simulink model "actual_flight"  (R2022a)
settings: Solver=ode4  StartTime=0.0  StopTime=10  FixedStep=0.001  RelTol=1e-3
InitFcn:
  | BeforeSim
undefined symbols (not defined in the file or in its folder): L_ref, S_ref
libraries: simulink_need_slupdate x12
settings Model: Creator=Hans  LastModifiedBy=24659
settings SolverCC: AlgebraicLoopSolver=TrustRegion
settings DataIOCC: ReturnWorkspaceOutputs=off
settings OptimizationCC: LifeSpan=inf
settings DebuggingCC: UnconnectedInputMsg=warning  UnconnectedOutputMsg=warning  UnconnectedLineMsg=warning  SFExecutionAtInitializationDiag=none  SFMachineParentedDataDiag=warning  ArithmeticOperatorsInVariantConditions=warning
settings HardwareCC: ProdBitPerSizeT=32  ProdBitPerPtrDiffT=32  ProdWordSize=32  ProdHWDeviceType=Specified
settings SFSimCC: SimUseLocalCustomCode=off  CustomCodeUndefinedFunction=UseInterfaceOnly
settings RTWCC: RTWUseLocalCustomCode=off
settings CodeAppCC: StateflowObjectComments=on

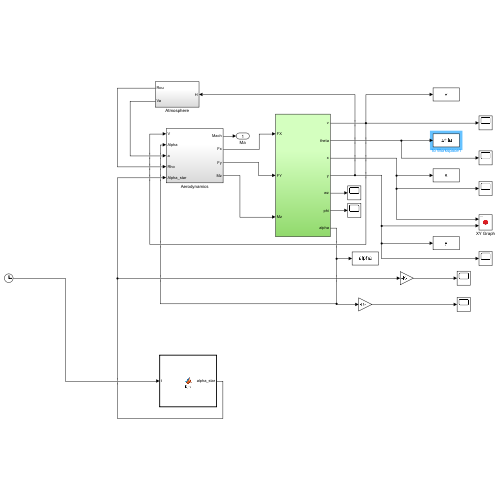
[thumbnail: Simulink's stored preview of the top-level diagram]
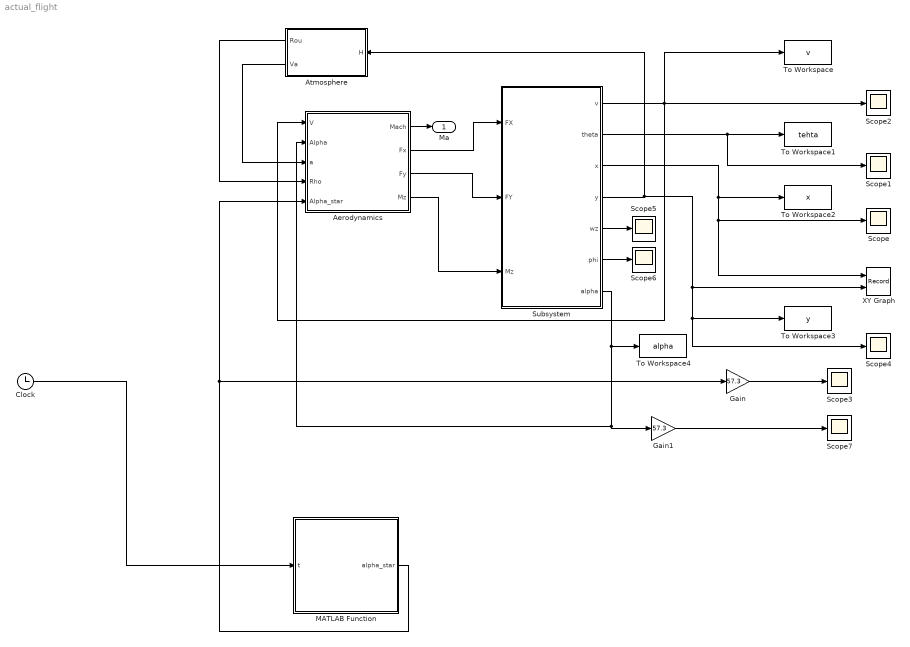
== system actual_flight ==
  Aerodynamics : Subsystem
  Atmosphere : Subsystem
  Clock : Clock
  Gain : Gain  Gain=57.3
  Gain1 : Gain  Gain=57.3
  MATLAB Function : MATLAB Function  TreatAsAtomicUnit=on
  Scope{,1..7} (8 alike) : Scope
  Subsystem : Subsystem
  To Workspace : ToWorkspace  VariableName=v  SaveFormat=Timeseries  SampleTime=-1
  To Workspace1 : ToWorkspace  VariableName=tehta  SaveFormat=Timeseries  SampleTime=-1
  To Workspace2 : ToWorkspace  VariableName=x  SaveFormat=Timeseries  SampleTime=-1
  To Workspace3 : ToWorkspace  VariableName=y  SaveFormat=Timeseries  SampleTime=-1
  To Workspace4 : ToWorkspace  VariableName=alpha  SaveFormat=Timeseries  SampleTime=-1
  XY Graph : Record  FileSettingsInternal="{\"entries\":[{\"content\":{\"excelSettings\":{\"content\":{},\"type\":\"Streamout.ExcelSettings\"}},\"type\":\"Streamout.FileSettingStorage\",\"uuid\":\"ac6b3081-8645-4955-ae6f-fd0c9016351f\"}],\"packageUris\":[\"http://schema.mathworks.com/mf0/streamout_blocks/R2020a\"],\"version\":\"1.0\"}"  Layout=[1 1]  SignalsInternal="{\"entries\":[{\"content\":{\"signals\":[{\"content\":{\"blockPath\":[\"actual_flight/XY Graph\"],\"channel\":[],\"dimensions\":[1],\"domain\":\"actual_flight/XY Graph\",\"lineColor\":\"#a2142f\",\"plots\":[1],\"port\":1,\"sid\":[\"\"],\"signalID\":117,\"signalName\":\"Subsystem:3\"},\"type\":\"RecordBlkView.Signal\",\"uuid\":\"a6b6c65e-2a84-4de5-9352-2b80d4c69f46\"},{\"content\":{\"blockPath\":[\"actual_flight/XY Graph\"],\"channel\":[],\"dimensions\":[1],\"domain\":\"actual_flight/XY Graph\",\"lineColor\":\"#139fff\",\"plots\":[1],\"port\":2,\"sid\":[\"\"],\"signalID\":121,\"signalName\":\"Subsystem:4\"},\"type\":\"RecordBlkView.Signal\",\"uuid\":\"7b7fe503-11ab-499b-9855-293f14eb9002\"}]},\"type\":\"RecordBlkView.InputSignals\",\"uuid\":\"3e16099a-8075-4753-8833-8a8d798b48ad\"}],\"packageUris\":[\"http://schema.mathworks.com/mf0/streamout_blocks/R2020a\"],\"version\":\"1.0\"}"  VisualizationBindings="{\"xyplotplugin\":{\"info\":[{\"series\":[{\"bindingParametersList\":[{\"parameter\":\"X-Axis\",\"signalID\":117,\"signalName\":\"Subsystem:3\"},{\"parameter\":\"Y-Axis\",\"signalID\":121,\"signalName\":\"Subsystem:4\"}],\"seriesID\":55315}],\"subplotID\":1}]}}"  CompatibilityTag=XY  st=-1
  Ma : Outport
  wires:
  Gain/1 -> Scope3/1
  Subsystem/4(y) -> To Workspace3/1, Scope4/1, XY Graph/2, Atmosphere/1(H)
  Subsystem/1(v) -> Aerodynamics/1(V), Scope2/1, To Workspace/1
  Aerodynamics/1(" Mach") -> Ma/1
  Aerodynamics/2(Fx) -> Subsystem/1(FX)
  Atmosphere/1(Rou) -> Aerodynamics/4(Rho)
  Aerodynamics/3(Fy) -> Subsystem/2(FY)
  Atmosphere/2(Va) -> Aerodynamics/3(a)
  Clock/1 -> MATLAB Function/1(t)
  Subsystem/2(theta) -> Scope1/1, To Workspace1/1
  Subsystem/3(x) -> XY Graph/1, Scope/1, To Workspace2/1
  MATLAB Function/1(alpha_star) -> Aerodynamics/5(Alpha_star), Gain/1
  Aerodynamics/4(" Mz") -> Subsystem/3(Mz)
  Subsystem/7(alpha) -> To Workspace4/1, Gain1/1, Aerodynamics/2(Alpha)
  Subsystem/5(wz) -> Scope5/1
  Subsystem/6(phi) -> Scope6/1
  Gain1/1 -> Scope7/1

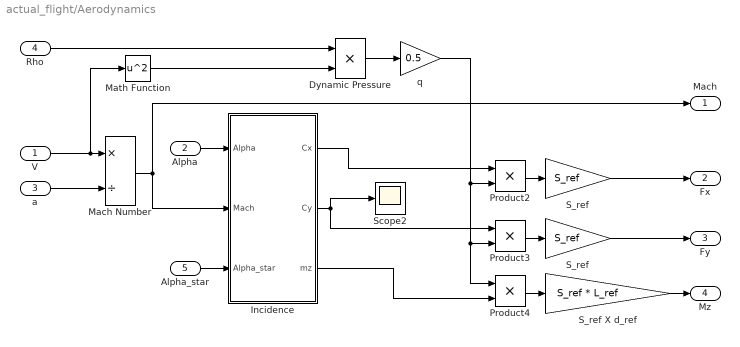
== system actual_flight/Aerodynamics ==
  V : Inport
  Alpha : Inport  Port=2
  a : Inport  Port=3
  Rho : Inport  Port=4
  Alpha_star : Inport  Port=5
  Dynamic Pressure : Product  InputSameDT=on  SaturateOnIntegerOverflow=on  OutDataTypeStr=Inherit: Same as first input
  Incidence : Subsystem
  Mach Number : Product  Inputs=*/  InputSameDT=on  SaturateOnIntegerOverflow=on  OutDataTypeStr=Inherit: Same as first input
  Math Function : Math  Operator=square  SignedPower=on
  Product2 : Product  InputSameDT=on  SaturateOnIntegerOverflow=on  OutDataTypeStr=Inherit: Same as first input
  Product3 : Product  InputSameDT=on  SaturateOnIntegerOverflow=on  OutDataTypeStr=Inherit: Same as first input
  Product4 : Product  InputSameDT=on  SaturateOnIntegerOverflow=on  OutDataTypeStr=Inherit: Same as first input
  S_ref : Gain  Gain=S_ref  SaturateOnIntegerOverflow=on  OutDataTypeStr=Inherit: Same as input  ParamDataTypeStr=Inherit: Same as input
  "S_ref " : Gain  Gain=S_ref  SaturateOnIntegerOverflow=on  OutDataTypeStr=Inherit: Same as input  ParamDataTypeStr=Inherit: Same as input
  S_ref X d_ref : Gain  Gain=S_ref * L_ref  SaturateOnIntegerOverflow=on  OutDataTypeStr=Inherit: Same as input  ParamDataTypeStr=Inherit: Same as input
  Scope2 : Scope
  q : Gain  Gain=0.5  SaturateOnIntegerOverflow=on  OutDataTypeStr=Inherit: Same as input  ParamDataTypeStr=Inherit: Same as input
  " Mach" : Outport  InitialOutput=0
  Fx : Outport  Port=2  InitialOutput=[0]
  Fy : Outport  Port=3  InitialOutput=0
  " Mz" : Outport  Port=4  InitialOutput=0
  wires:
  Incidence/2(Cy) -> Product3/1, Scope2/1
  Product3/1 -> "S_ref "/1
  S_ref/1 -> Fx/1
  "S_ref "/1 -> Fy/1
  V/1 -> Math Function/1, Mach Number/1
  Product2/1 -> S_ref/1
  Mach Number/1 -> " Mach"/1, Incidence/2(Mach)
  Incidence/3(mz) -> Product4/2
  Product4/1 -> S_ref X d_ref/1
  a/1 -> Mach Number/2
  S_ref X d_ref/1 -> " Mz"/1
  q/1 -> Product2/2, Product3/2, Product4/1
  Rho/1 -> Dynamic Pressure/1
  Dynamic Pressure/1 -> q/1
  Math Function/1 -> Dynamic Pressure/2
  Incidence/1(Cx) -> Product2/1
  Alpha/1 -> Incidence/1(Alpha)
  Alpha_star/1 -> Incidence/3(Alpha_star)

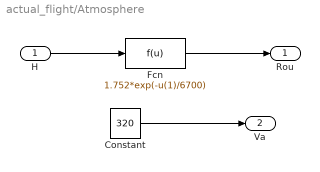
== system actual_flight/Atmosphere ==
  H : Inport
  Constant : Constant  Value=320
  Fcn : Fcn  Expr=1.752*exp(-u(1)/6700)
  Rou : Outport
  Va : Outport  Port=2
  wires:
  H/1 -> Fcn/1
  Fcn/1 -> Rou/1
  Constant/1 -> Va/1

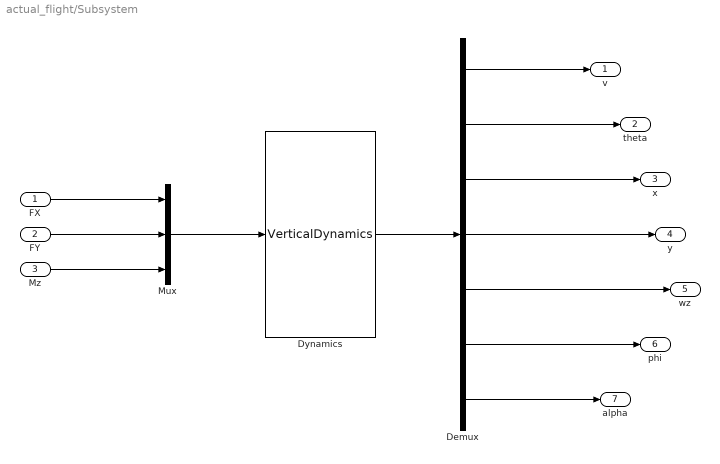
== system actual_flight/Subsystem ==
  FX : Inport
  FY : Inport  Port=2
  Mz : Inport  Port=3
  Demux : Demux  Outputs=7
  Dynamics : S-Function  FunctionName=VerticalDynamics  SFunctionDeploymentMode=off  EnableBusSupport=off
  Mux : Mux  Inputs=3
  v : Outport
  theta : Outport  Port=2
  x : Outport  Port=3
  y : Outport  Port=4
  wz : Outport  Port=5
  phi : Outport  Port=6
  alpha : Outport  Port=7
  wires:
  FX/1 -> Mux/1
  FY/1 -> Mux/2
  Mux/1 -> Dynamics/1
  Dynamics/1 -> Demux/1
  Demux/1 -> v/1
  Demux/2 -> theta/1
  Demux/3 -> x/1
  Demux/4 -> y/1
  Mz/1 -> Mux/3
  Demux/5 -> wz/1
  Demux/6 -> phi/1
  Demux/7 -> alpha/1

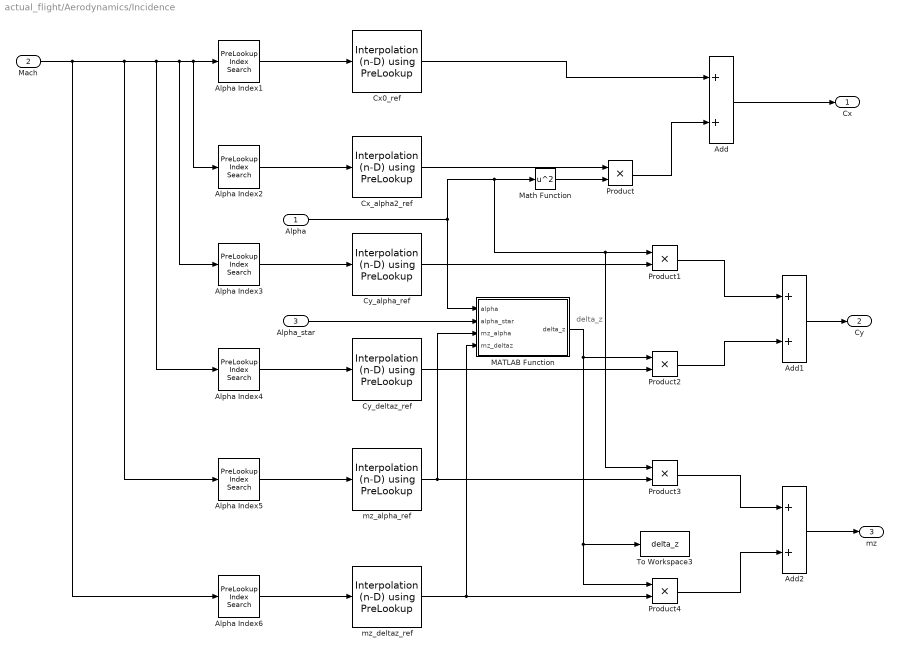
== system actual_flight/Aerodynamics/Incidence ==
  note: delta_z
  Alpha : Inport
  Mach : Inport  Port=2
  Alpha_star : Inport  Port=3
  Add : Sum
  Add1 : Sum
  Add2 : Sum
  Alpha Index{1..6} (6 alike) : simulink_need_slupdate/PreLookup Index Search  bpData=Mach_ref  searchMode=Binary Search  cacheBpFlag=on  outputFlag=off  IndexDataType=uint32  extrapMode=Linear Extrapolation  rangeErrorMode=None
      settings: SourceProductBaseCode=SL
  Cx0_ref : simulink_need_slupdate/Interpolation (n-D) using PreLookup  numDimsPopupSelect=1  explicitNumDims=2  table=Cx0_ref  interpMethod=Linear  extrapMethod=Linear  rangeErrorMode=None  NumSelectionDims=0
      settings: SourceProductBaseCode=SL
  Cx_alpha2_ref : simulink_need_slupdate/Interpolation (n-D) using PreLookup  numDimsPopupSelect=1  explicitNumDims=2  table=Cx_alpha2_ref  interpMethod=Linear  extrapMethod=Linear  rangeErrorMode=None  NumSelectionDims=0
      settings: SourceProductBaseCode=SL
  Cy_alpha_ref : simulink_need_slupdate/Interpolation (n-D) using PreLookup  numDimsPopupSelect=1  explicitNumDims=2  table=Cy_alpha_ref  interpMethod=Linear  extrapMethod=Linear  rangeErrorMode=None  NumSelectionDims=0
      settings: SourceProductBaseCode=SL
  Cy_deltaz_ref : simulink_need_slupdate/Interpolation (n-D) using PreLookup  numDimsPopupSelect=1  explicitNumDims=2  table=Cy_deltaz_ref  interpMethod=Linear  extrapMethod=Linear  rangeErrorMode=None  NumSelectionDims=0
      settings: SourceProductBaseCode=SL
  MATLAB Function : MATLAB Function  TreatAsAtomicUnit=on
  Math Function : Math  Operator=square  SignedPower=on
  Product{,1..4} (5 alike) : Product
  To Workspace3 : ToWorkspace  VariableName=delta_z  SaveFormat=Timeseries  SampleTime=-1
  mz_alpha_ref : simulink_need_slupdate/Interpolation (n-D) using PreLookup  numDimsPopupSelect=1  explicitNumDims=2  table=mz_alpha_ref  interpMethod=Linear  extrapMethod=Linear  rangeErrorMode=None  NumSelectionDims=0
      settings: SourceProductBaseCode=SL
  mz_deltaz_ref : simulink_need_slupdate/Interpolation (n-D) using PreLookup  numDimsPopupSelect=1  explicitNumDims=2  table=mz_deltaz_ref  interpMethod=Linear  extrapMethod=Linear  rangeErrorMode=None  NumSelectionDims=0
      settings: SourceProductBaseCode=SL
  Cx : Outport  InitialOutput=0
  Cy : Outport  Port=2  InitialOutput=0
  mz : Outport  Port=3  InitialOutput=0
  wires:
  Alpha Index1/1 -> Cx0_ref/1
  Alpha Index2/1 -> Cx_alpha2_ref/1
  Alpha Index3/1 -> Cy_alpha_ref/1
  Alpha Index4/1 -> Cy_deltaz_ref/1
  Alpha Index5/1 -> mz_alpha_ref/1
  Alpha Index6/1 -> mz_deltaz_ref/1
  Mach/1 -> Alpha Index6/1, Alpha Index5/1, Alpha Index4/1, Alpha Index3/1, Alpha Index2/1, Alpha Index1/1
  Cx_alpha2_ref/1 -> Product/1
  Alpha/1 -> Product3/1, Product1/1, Math Function/1, MATLAB Function/1(alpha)
  Math Function/1 -> Product/2
  Cx0_ref/1 -> Add/1
  Product/1 -> Add/2
  Add/1 -> Cx/1
  Cy_alpha_ref/1 -> Product1/2
  MATLAB Function/1(delta_z) -> Product4/1, To Workspace3/1, Product2/1
  Cy_deltaz_ref/1 -> Product2/2
  Product1/1 -> Add1/1
  Product2/1 -> Add1/2
  Add1/1 -> Cy/1
  mz_alpha_ref/1 -> MATLAB Function/3(mz_alpha), Product3/2
  mz_deltaz_ref/1 -> MATLAB Function/4(mz_deltaz), Product4/2
  Product3/1 -> Add2/1
  Product4/1 -> Add2/2
  Add2/1 -> mz/1
  Alpha_star/1 -> MATLAB Function/2(alpha_star)

== matlab function actual_flight/Aerodynamics/Incidence/MATLAB Function ==
  data: alpha input; delta_z output; alpha_star input; mz_alpha input; mz_deltaz input
function delta_z = fcn(alpha,alpha_star,mz_alpha,mz_deltaz)
K = 1.0;
delta_zB = -mz_alpha*alpha_star/mz_deltaz;
delta_z = delta_zB + K*(alpha-alpha_star);

== matlab function actual_flight/MATLAB Function ==
  data: t input; alpha_star output
function alpha_star = fcn(t)
alpha_star_tem = 0;
if t > 0 && t < 3
    alpha_star_tem = 0;
else
    alpha_star_tem = 5;
end
alpha_star = alpha_star_tem*pi/180;%将度转换为弧度
